simulink model "sldemo_fuelsys_dd_org"  (Simulink 10.0)
settings: Solver=ode45  StartTime=0.0  StopTime=2000  FixedStep=0.001  RelTol=1e-5  AbsTol=1e-6
libraries: simulink x2
Description:
  | This is a model of a fuel control system where Stateflow(R) is used to handle the fault management of the system.
  | The system contains four separate sensors: a throttle sensor, a speed sensor, an oxygen sensor, and a pressure sensor.
  | Each of these sensors is represented by a parallel state in Stateflow.  Each parallel state contains two substates, a
  | normal state and a failed state (the exception being the oxygen sensor, which also contains a warmup state).
  | 
  | If any of the sensor readings is outside an acceptable range, then a fault is registered in Stateflow, and the
  | substate of the corresponding subsystem transitions to the failed state.  If a subsystem recovers, it can
  | transition back to the normal state.  The number of failures in the system at any given time is represented
  | in the Sens_Failure_Counter parallel state.
  | 
  | The last parallel state in the Stateflow chart is called Fueling_Mode.  This state regulates the oxygen to
  | fuel mixture ratio.  If a failure is detected, then the oxygen to fuel ratio is increased.  If multiple failures
  | are detected, then the fuel system is disabled until there are no longer multiple failures in the system.
CloseFcn:
  | clear sldemo_fuelsys_output
settings Model: DataDictionary=sldemo_fuelsys_dd.sldd  EnableAccessToBaseWorkspace=off  Creator=The MathWorks, Inc.  LastModifiedBy=bhisma  ExtModeTrigMode=oneshot  ExtModeArmWhenConnect=off  ExtModeAutoUpdateStatusClock=off
settings SolverCC: AutoScaleAbsTol=off
settings DataIOCC: SaveFormat=StructureWithTime  SaveOutput=off  SaveTime=off  SignalLoggingName=sldemo_fuelsys_output
settings OptimizationCC: DefaultParameterBehavior=Inlined  UseDivisionForNetSlopeComputation=UseDivisionForReciprocalsOfIntegersOnly  InlineInvariantSignals=on  EnhancedBackFolding=on  StrengthReduction=on  BooleansAsBitfields=on  PassReuseOutputArgsAs=Individual arguments  ExpressionDepthLimit=2147483647  StateBitsets=on  DataBitsets=on  ZeroExternalMemoryAtStartup=off  ZeroInternalMemoryAtStartup=off  NoFixptDivByZeroProtection=on  EfficientFloat2IntCast=on  LifeSpan=1  EfficientTunableParamExpr=on
settings DebuggingCC: SignalInfNanChecking=error  AlgebraicLoopMsg=none  SaveWithParameterizedLinksMsg=none  MergeDetectMultiDrivingBlocksExec=error  CheckExecutionContextPreStartOutputMsg=on  CheckExecutionContextRuntimeOutputMsg=on  IntegerOverflowMsg=none  ParameterDowncastMsg=warning  ParameterOverflowMsg=none  ParameterPrecisionLossMsg=none  UnderSpecifiedDataTypeMsg=warning  FcnCallInpInsideContextMsg=warning  UniqueDataStoreMsg=error  BusObjectLabelMismatch=error  AllowSymbolicDim=off  StateNameClashWarn=warning  StrictBusMsg=ErrorOnBusTreatedAsVector  IntegerSaturationMsg=none
settings HardwareCC: ProdIntDivRoundTo=Zero  ProdEndianess=LittleEndian  ProdHWDeviceType=Specified
settings SFSimCC: SimParseCustomCode=off  MATLABDynamicMemAlloc=off
settings RTWCC: Description=Real-Time Workshop Embedded Coder  SystemTargetFile=ert.tlc  TemplateMakefile=ert_default_tmf  GenerateReport=on  RTWVerbose=off  IncludeHyperlinkInReport=on  LaunchReport=on  GenerateTraceInfo=on  GenerateTraceReport=on  GenerateTraceReportSl=on  GenerateTraceReportSf=on  GenerateTraceReportEml=on
settings CodeAppCC: ForceParamTrailComments=on  IgnoreCustomStorageClasses=off  IgnoreTestpoints=on  SimulinkDataObjDesc=on  SFDataObjDesc=on  CustomSymbolStrGlobalVar=rt$N$M  CustomSymbolStrType=$N$M  CustomSymbolStrFcn=$N$M$F  CustomSymbolStrMacro=$N$M  InsertBlockDesc=on  InternalIdentifier=Classic  ReqsInCode=on
settings ERTTargetCC: MultiwordLength=2048  GenerateSampleERTMain=on  IncludeMdlTerminateFcn=off  SupportAbsoluteTime=off  SupportNonFinite=off  SupportComplex=off  InlinedParameterPlacement=NonHierarchical  ERTCustomFileTemplate=example_file_process.tlc  ConvertIfToSwitch=off  SuppressUnreachableDefaultCases=off
settings ConfigComp: CovScope=ReferencedModels  CovIncludeTopModel=off  CovModelRefExcluded=sldemo_fuelsys_dd_plant  CovExternalEMLEnable=off  CovSFcnEnable=off

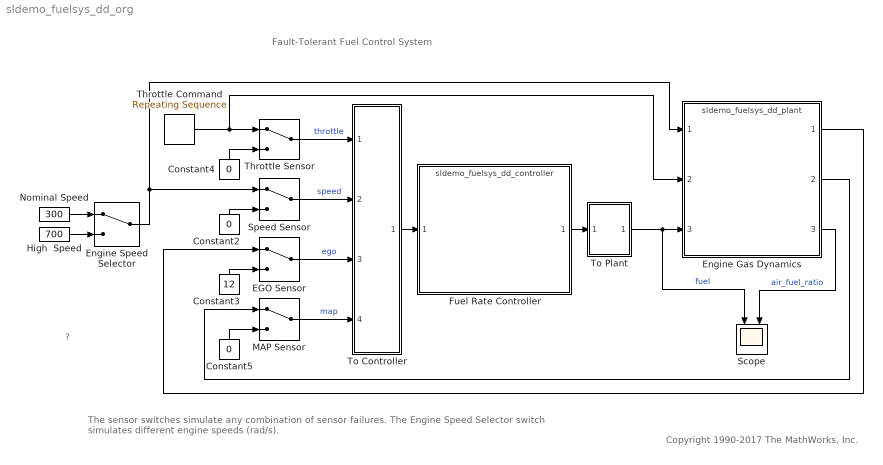
== system sldemo_fuelsys_dd_org ==
  note: Fault-Tolerant Fuel Control System
  note: Copyright 1990-2017 The MathWorks, Inc.
  note: The sensor switches simulate any combination of sensor failures.
      | The Engine Speed Selector switch simulates different engine speeds (rad/s).
  note: ?
  Constant2 : Constant  Value=0
  Constant3 : Constant  Value=12
  Constant4 : Constant  Value=0
  Constant5 : Constant  Value=0
  EGO Sensor : ManualSwitch
  Engine Speed Selector : ManualSwitch
  Engine Gas Dynamics : ModelReference  ModelNameDialog=sldemo_fuelsys_dd_plant.slx  SimulationMode=Normal  ModelReferenceVersion=1.551
  Fuel Rate Controller : ModelReference  ModelNameDialog=sldemo_fuelsys_dd_controller.slx  SimulationMode=Normal  ModelReferenceVersion=1.560
  High  Speed : Constant  Value=700
  MAP Sensor : ManualSwitch
  Nominal Speed : Constant  Value=300
  Scope : Scope  NumInputPorts=2
  Speed Sensor : ManualSwitch
  Throttle Command : simulink/Sources/Repeating Sequence  rep_seq_t=[0 2 4]  rep_seq_y=[10 20 10]
  Throttle Sensor : ManualSwitch
  To Controller : Subsystem
      mask Display: fprintf('Convert')
  To Plant : Subsystem
      mask Display: fprintf('Convert')
  wires:
  Engine Gas Dynamics/3 -> Scope/2  "air_fuel_ratio"
  Engine Speed Selector/1 -> Engine Gas Dynamics/1, Speed Sensor/1
  Fuel Rate Controller/1 -> To Plant/1(In1)
  Engine Gas Dynamics/1 -> EGO Sensor/1
  Constant5/1 -> MAP Sensor/2
  Constant3/1 -> EGO Sensor/2
  Throttle Command/1 -> Engine Gas Dynamics/2, Throttle Sensor/1
  Constant2/1 -> Speed Sensor/2
  Constant4/1 -> Throttle Sensor/2
  Engine Gas Dynamics/2 -> MAP Sensor/1
  High  Speed/1 -> Engine Speed Selector/2
  Nominal Speed/1 -> Engine Speed Selector/1
  EGO Sensor/1 -> To Controller/3(ego)  "ego"
  MAP Sensor/1 -> To Controller/4(map)  "map"
  Throttle Sensor/1 -> To Controller/1(throttle)  "throttle"
  Speed Sensor/1 -> To Controller/2(speed)  "speed"
  To Plant/1(Out1) -> Scope/1, Engine Gas Dynamics/3  "fuel"
  To Controller/1(sensors) -> Fuel Rate Controller/1

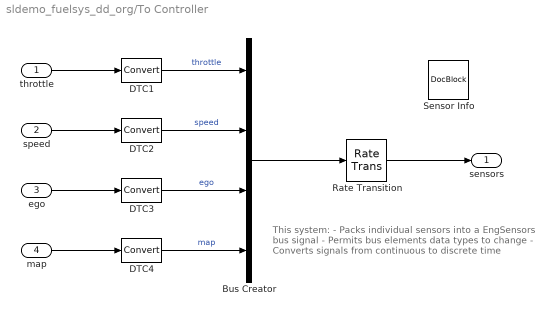
== system sldemo_fuelsys_dd_org/To Controller ==
  note: This system:
      | - Packs individual sensors into a EngSensors bus signal
      | - Permits bus elements data types to change
      | - Converts signals from continuous to discrete time
  throttle : Inport
  speed : Inport  Port=2
  ego : Inport  Port=3
  map : Inport  Port=4
  Bus Creator : BusCreator  Inputs=4  OutDataTypeStr=Bus: EngSensors  NonVirtualBus=on
  DTC{1..4} (4 alike) : DataTypeConversion  SampleTime=[0 1]
  Rate Transition : RateTransition  OutPortSampleTime=0.01
  Sensor Info : simulink/Model-Wide Utilities/DocBlock  DocumentType=Text
      content=|
      | Measurement Descriptions
      | ========================
      |
      | Throttle Angle (degrees):
      | min=3, max=90, precision=0.1
      |
      | Engine Speed (radians/sec.):
      | min=0, max=620, precision=.1
      |
      | Ego Sensor (volts):
      | min=0, max=12, precision=.05
      |
      | Manifold Pressure (bar):
      | min=0.001, max=1, precision=.001
  sensors : Outport  VectorParamsAs1DForOutWhenUnconnected=off
  wires:
  throttle/1 -> DTC1/1
  DTC1/1 -> Bus Creator/1  "throttle"
  speed/1 -> DTC2/1
  DTC2/1 -> Bus Creator/2  "speed"
  ego/1 -> DTC3/1
  DTC3/1 -> Bus Creator/3  "ego"
  map/1 -> DTC4/1
  DTC4/1 -> Bus Creator/4  "map"
  Bus Creator/1 -> Rate Transition/1
  Rate Transition/1 -> sensors/1

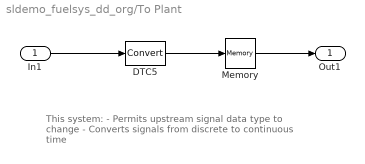
== system sldemo_fuelsys_dd_org/To Plant ==
  note: This system:
      | - Permits upstream signal data type to change
      | - Converts signals from discrete to continuous time
  In1 : Inport
  DTC5 : DataTypeConversion
  Memory : Memory
  Out1 : Outport  VectorParamsAs1DForOutWhenUnconnected=off
  wires:
  In1/1 -> DTC5/1
  DTC5/1 -> Memory/1
  Memory/1 -> Out1/1
